simulink model "ds_modelica_weathercsv"  (R2020a)
settings: Solver=ode1  StartTime=0.0  StopTime=24*3600  FixedStep=0.001  RelTol=1e-3
PostLoadFcn:
  | if any(exist('dsrtsu_mdlpostloadfcn', 'file') ~= 0), dsrtsu_mdlpostloadfcn('Execute', bdroot); end
InitFcn:
  | , if any(exist('rtifpga_mdlclblib', 'file') ~= 0), rtifpga_mdlclblib('Init', bdroot); end,
  | , if any(exist('dsmpb_private', 'file') ~= 0), dsmpb_private('dsmpb_mdlclblib', 'Init', bdroot); end,
libraries: dsmpblib x1
PreSaveFcn:
  | , if any(exist('dsmpb_private', 'file') ~= 0), dsmpb_private('dsmpb_mdlclblib', 'PreSave', bdroot); end,
CloseFcn:
  | , if any(exist('dsmpb_private', 'file') ~= 0), dsmpb_private('dsmpb_mdlclblib', 'Close', bdroot); end,
settings Model: RTICANMMDATA=struct('GeneralSetupData',struct('modelroot','D:\github\dspace-modelica-example\dSpaceExample','generalsettings',struct('filesettings',struct('destfolder',struct('Name','RTICANMM_FILES','Check',1),'buildfolder',struct('Name','.','Check',1),'AbsDestfolder',struct('Name','D:\github\dspace-modelica-example\dSpaceExample\RTICANMM_FILES'),'AbsBuildfolder',struct('Name','D:\github\dspace-modelica-example\dSpaceExample'))),'options',struct('addpaths',1,'rmpaths',1,'addtrcexclusion',true,'cannavigator',struct('checkmonitoring',0),'show_usrtrc',0,'use_usrtrc',0),'advanced',struct('options',ones(1,100)),'MPSetup',{{}},'RTI',struct('Type','DSRT','Ver','4.3','Date','02-May-2020'),'modelname','ds_modelica_weathercsv','block','ds_modelica_weathercsv'))  DSRTSU_INTERNAL_RTIFPGA=160  DSMPB_ID_DATA={'153',struct('BlockId','811b07df-2fcb-4c14-ad4d-f777e9630052','SignalIds',{{'eb3c2c6c-56b8-4259-a6b1-e5e06496ac5b'}})}  Creator=yangyang.fu  LastModifiedBy=yangyang.fu
settings OptimizationCC: BlockReduction=off  ConditionallyExecuteInputs=off  OptimizeBlockIOStorage=off  BufferReuse=off
settings DebuggingCC: TasksWithSamePriorityMsg=none
settings HardwareCC: ProdBitPerPointer=32  ProdBitPerSizeT=32  ProdBitPerPtrDiffT=32  ProdLargestAtomicInteger=Integer  ProdWordSize=32  ProdLongLongMode=on  ProdHWDeviceType=Custom Processor->Custom
settings ModelReferenceCC: EnableParallelModelReferenceBuilds=on
settings SFSimCC: MATLABDynamicMemAlloc=off
settings RTWCC: Description=dSPACE Run-Time Target (for VEOS on Windows and ConfigurationDesk)  SystemTargetFile=dsrt.tlc  GenCodeOnly=on  MakeCommand=make_dsrt  TemplateMakefile=dsrt_default_tmf  RTWVerbose=off  CustomInclude="\"C:\\Program Files\\Dymola 2021\\Source\" \"D:\\github\\dspace-modelica-example\\Libraries\\Buildings 7.0.0\\Resources\\C-Sources\""
settings STFCustomTargetCC: TargetLangStandard=C99 (ISO)  ParMdlRefBuildCompliant=on  SystemTargetFile=dsrt.tlc
settings GRTTargetCC: CompOptLevelCompliant=off  ConcurrentExecutionCompliant=off  CombineOutputUpdateFcns=off  MatFileLogging=off  CPPClassGenCompliant=off  UseToolchainInfoCompliant=off

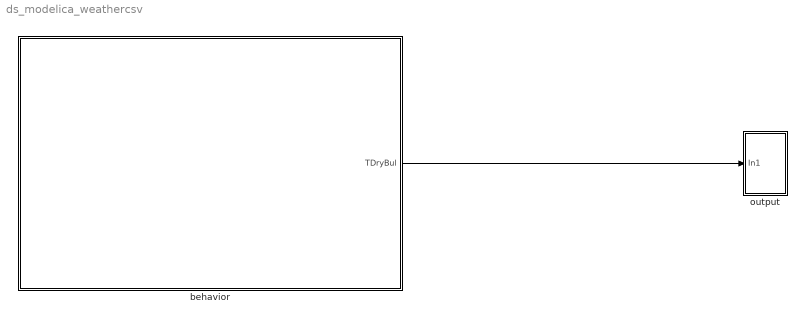
== system ds_modelica_weathercsv ==
  behavior : Subsystem
  output : Subsystem
  wires:
  behavior/1(TDryBul) -> output/1(In1)

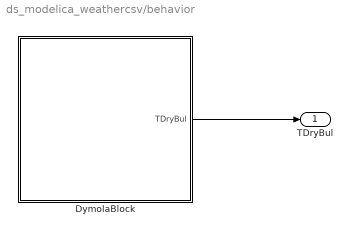
== system ds_modelica_weathercsv/behavior ==
  DymolaBlock : Subsystem  Tag=20-Oct-2021 17:35:29#975
      mask help:
      | Dymola block.
      | A dymola block allows acausal physical modeling.
      | See Dymola manual for usage.
      settings: CopyFcn=newDymolaGui('20-Oct-2021 17:35:29#975','Copy');  DeleteFcn=if exist('newDymolaGui') newDymolaGui('ds_modelica_weathercsv/behavior/DymolaBlock','Delete'); end;  NameChangeFcn=newDymolaGui('20-Oct-2021 17:35:29#975','Copy');  OpenFcn=newDymolaGui('ds_modelica_weathercsv/behavior/DymolaBlock','Init');
      mask Display: image(reshape([1;1;1;1;1;1;1;1;1;1;1;1;1;1;1;1;1;1;1;1;1;1;0;0;0;0;0;0;0;0;0;0;1;1;1;1;1;1;1;1;0;1;1;1;1;1;1;1;1;0;1;1;1;1;1;0;0;0;0;0;0;0;1;1;0;0;0;0;0;0;0;1;1;0;0;0;0;0;0;0;1;1;0;0;0;0;0;0;0;1;1;0;0;0;0;0;0;0;1;1;0;0;0;0;0;0;0;1;1;0;0;0;0;0;0;0;1;1;0;0;0;0;0;0;0;1;1;0;0;0;0;0;0;0;1;1;0;0;0;0;0;0;0;1;1;0;0;0;0;0;0;0;1;1;0;0;0;0;0;0;0;1;1;0;0;0;0;0;0;0;1;1;0;0;0;0;0;0;0;1;1;0;0;0;0;0;0;0;1;1;0;0;0;0;0;0;0;1;1;0;0;0;0;0;0;0;1;1;0;0;0;0;0;0;0;1;1;0;0;0;0;0;0;0;1;1;0;0;0;0;0;0;0;1;1;0;0;0;0;0;0;0;1;1;0;0;0;0;0;0;0;1;1;0;0;0;0;0;0;0;1;1;0;0;0;0;0;0;0;1;1;1;1;1;0;1;1;1;1;1;1;1;1;0;1;1;1;1;1;1;1;1;0;0;0;0;0;0;0;0;0;0;1;1;1;1;1;1;1;1;1;1;1;1;1;1;1;1;1;1;1;1;1;1;1;1;1;1;1;1;1;1;1;1;1;1;1;1;1;1;1;1;1;1;1;1;0;0;0;0;0;0;0;0;0;0;1;1;1;1;1;1;1;1;0;1;1;1;1;1;1;1;1;0;1;1;1;1;1;0;0;0;0;0;0;0;1;1;0;0;0;0;0;0;0;1;1;0;0;0;0;0;0;0;1;1;0;0;0;0;0;0;0;1;1;0;0;0;0;0;0;0;1;1;0;0;0;0;0;0;0;1;1;0;0;0;0;0;0;0;1;1;0;0;0;0;0;0;0;1;1;0;0;0;0;0;0;0;1;1;0;0;0;0;0;0;0;1;1;0;0;0;0;0;0;0;1;1;0;0;0;0;0;0;0;1;1;0;0;0;0;0;0;0;1;1;0;0;0;0;0;0;0;1;1;0;0;0;0;0;0;0;1;1;0;0;0;0;0;0;0;1;1;0;0;0;0;0;0;0;1;1;0;0;0;0;0;0;0;1;1;0;0;0;0;0;0;0;1;1;0;0;0;0;0;0;0;1;1;0;0;0;0;0;0;0;1;1;0;0;0;0;0;0;0;1;1;0;0;0;0;0;0;0;1;1;0;0;0;0;0;0;0;1;1;1;1;1;0;1;1;1;1;1;1;1;1;0;1;1;1;1;1;1;1;1;0;0;0;0;0;0;0;0;0;0;1;1;1;1;1;1;1;1;1;1;1;1;1;1;1;1;1;1;1;1;1;1;1;1;1;1;1;1;1;1;1;1;1;1;1;1;1;1;1;1;1;1;1;1;0;0;0;0;0;0;0;0;0;0;1;1;1;1;1;1;1;1;0;1;1;1;1;1;1;1;1;0;1;1;1;1;1;0;0;0;0;0;0;0;1;1;0;0;0;0;0;0;0;1;1;0;1;1;1;1;1;0;1;1;0;1;1;1;1;1;0;1;1;0;1;1;1;1;1;0;1;1;0;1;1;1;1;1;0;1;1;0;1;1;1;1;1;0;1;1;0;1;1;1;1;1;0;1;1;0;1;1;1;1;1;0;1;1;0;1;1;1;1;1;0;1;1;0;1;1;1;1;1;0;1;1;0;1;1;1;1;1;0;1;1;0;1;1;1;1;1;0;1;1;0;1;1;1;1;1;0;1;1;0;1;1;1;1;1;0;1;1;0;1;1;1;1;1;0;1;1;0;1;1;1;1;1;0;1;1;0;1;1;1;1;1;0;1;1;0;1;1;1;1;1;0;1;1;0;1;1;1;1;1;0;1;1;0;1;1;1;1;1;0;1;1;0;1;1;1;1;1;0;1;1;0;0;0;0;0;0;0;1;1;0;0;0;0;0;0;0;1;1;1;1;1;0;1;1;1;1;1;1;1;1;0;1;1;1;1;1;1;1;1;0;0;0;0;0;0;0;0;0;0;1;1;1;1;1;1;1;1;1;1;1;1;1;1;1;1;1;1;1;1;1;1],18,18,3),[.2,.2,.6,.6])
  TDryBul : Outport
  wires:
  DymolaBlock/1(TDryBul) -> TDryBul/1

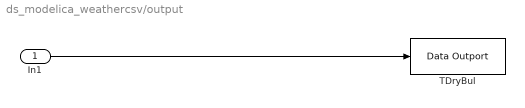
== system ds_modelica_weathercsv/output ==
  In1 : Inport
  TDryBul : dsmpblib/Data Outport  Priority=-10000
      settings: SourceProductName=dSPACE Model Interface Blockset
  wires:
  In1/1 -> TDryBul/1

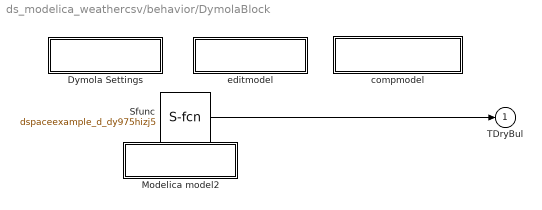
== system ds_modelica_weathercsv/behavior/DymolaBlock ==
  Dymola Settings : Subsystem  mask{ModelName=dSpaceExample.Debug.WeatherFromCSV, MoFileName=D:/github/dspace-modelica-example/dSpaceExample/Debug/WeatherFromCSV.mo, dSpace=, BusConnector=[], ResultFile=[], ResultFileOnline=[], ResultDt=[], Libs=:, bigobj=[], ImportFolder=[], guimode=[], ModelName2=[], forRuntime=[], MEXLoad=[], omitDescription=[], ResultName=dspaceexample_d_dy975hizj5}
      mask prompts: ModelName "Name of Dymola model"; MoFileName "File Name (including .mo)"; ResultFile "Create Result"; ResultFileOnline "Load result"; ResultDt "Result min dt"; Libs "Used Libraries"; bigobj "Compiler flag /bigobj"; ImportFolder "Import folder"; guimode "GUI mode flag"; ModelName2 "Model name for import mode"; forRuntime "Runtime export"; MEXLoad "Compiled S-function"; omitDescription "Omit description strings"; ResultName "Name of result file"
      mask Display: disp('Dymola Settings');
  Modelica model2 : Subsystem
      mask Display: disp('Change parameters');
  Sfunc : S-Function  Tag=975hizj5  FunctionName=dspaceexample_d_dy975hizj5  Parameters=[timTab_verboseRead;timTab_offset;timTab_startTime;timTab_timeEvents],[]  PortCounts=[0;1]  SFunctionDeploymentMode=off  EnableBusSupport=off  mask{timTab_verboseRead=1, timTab_offset=0, timTab_startTime=0, timTab_timeEvents=1}
      mask prompts: timTab_verboseRead "timTab.verboseRead"; timTab_offset "timTab.offset"; timTab_startTime "timTab.startTime"; timTab_timeEvents "timTab.timeEvents"
      mask Display: image(imread('Dymola.bmp'))
  compmodel : Subsystem
      settings: OpenFcn=compileModelica('ds_modelica_weathercsv/behavior/DymolaBlock');
      mask Display: disp('Compile Modelica model');
  editmodel : Subsystem
      settings: OpenFcn=editModelica('ds_modelica_weathercsv/behavior/DymolaBlock');
      mask Display: disp('Edit Modelica model');
  TDryBul : Outport
  wires:
  Sfunc/1 -> TDryBul/1

== system ds_modelica_weathercsv/behavior/DymolaBlock/Dymola Settings ==

== system ds_modelica_weathercsv/behavior/DymolaBlock/Modelica model2 ==

== system ds_modelica_weathercsv/behavior/DymolaBlock/compmodel ==

== system ds_modelica_weathercsv/behavior/DymolaBlock/editmodel ==
